simulink model "HydroPower"  (R2024b)
settings: Solver=ode4  StartTime=0.0  StopTime=200  FixedStep=0.001  RelTol=1e-3
values from neighbouring files (symbols this model uses):
  Af = 0.01    [Data__MOTOR.m]    (also in Generator_Data.m = 0.0001; Generator_Datatest.m)
  Bf = 0.0002    [Data__MOTOR.m]    (also in Generator_Data.m = 2e-05; Generator_Datatest.m)
  Cr = 0    [Generator_Data.m]
  CurrentFaultSwitch = 0    [Data__MOTOR.m]    (also in Generator_Data.m = 1; Generator_Datatest.m)
  f = 0.001    [Data__MOTOR.m]    (also in Generator_Data.m = 0)
  J = 0.0012    [Data__MOTOR.m]    (also in Generator_Data.m = 0.263; Generator_Datatest.m = 0.263)
  Ld = 1.4e-3+L_charge    (= 0.0014)    [Generator_Data.m]    (also in Generator_Datatest.m = 0.0231)
  Lq = 2.8e-3+L_charge    (= 0.0028)    [Generator_Data.m]    (also in Generator_Datatest.m = 0.0231)
  P = 4    [Generator_Data.m]    (also in Generator_Datatest.m = 3)
  Phif = 0.8    [Generator_Data.m]
  rate_noise_i = 0.02*In    (= 0.22)    [Data__MOTOR.m]    (also in Generator_Data.m = 0.02; Generator_Datatest.m)
  rate_noise_w = 0.02*Wn    (= 2.96)    [Data__MOTOR.m]    (also in Generator_Data.m = 0.002; Generator_Datatest.m)
  Rs = 0.6+R_charge    (= 0.6)    [Generator_Data.m]    (also in Generator_Datatest.m = 0.48)
  StartStop = 0    [Data__MOTOR.m]    (also in Generator_Data.m; Generator_Datatest.m)
  Te = 0.1    [Data__MOTOR.m]    (also in Generator_Data.m = 1; Generator_Datatest.m)
  Vd = 0    [Generator_Data.m]
  VelocityFaultSwitch = 0    [Data__MOTOR.m]    (also in Generator_Data.m = 1; Generator_Datatest.m)
  Vq = 0    [Generator_Data.m]
  wm = 2*pi*50/P    (= 78.5398163397)    [Generator_Data.m]
undefined symbols (not defined in the file or in its folder): dspblkCoreblockFVToolHelper, gcbh
libraries: SignalEditorBlockLib x3
(part 3 of 3)

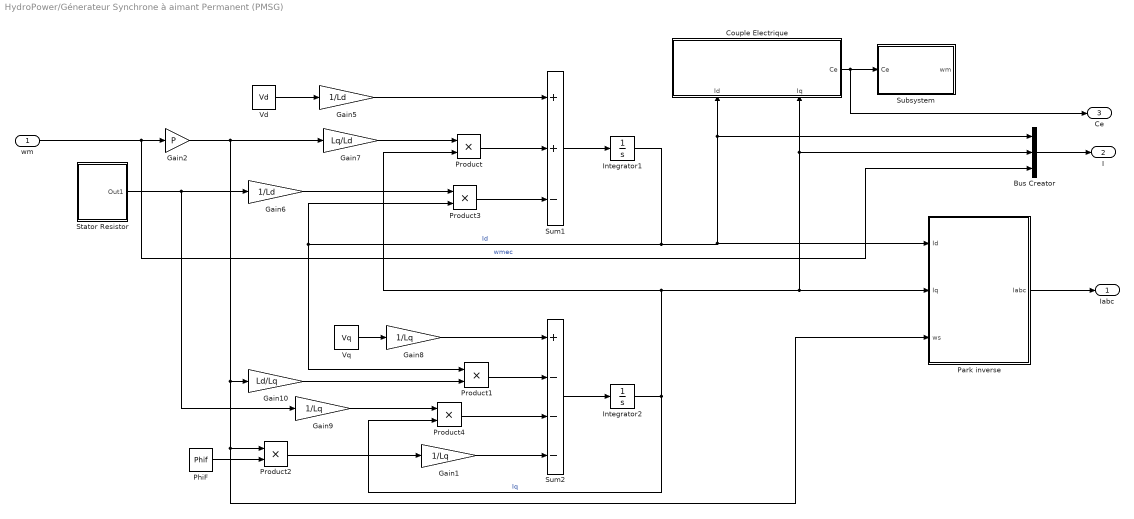
== system HydroPower/Génerateur Synchrone à aimant Permanent (PMSG) ==
  "wm " : Inport
  Bus Creator : BusCreator  Inputs=3
  Couple Electrique : Subsystem
      settings: PortSchema="{\"entries\":[{\"content\":{\"sides\":[{\"content\":{},\"type\":\"ConnectorPlacement.EquallySpacedRectSide\",\"uuid\":\"d44e9c0e-d895-4bd1-ae10-379ff1646526\"},{\"content\":{\"connectorIds\":[\"Out1\"],\"side\":\"RIGHT\"},\"type\":\"ConnectorPlacement.EquallySpacedRectSide\",\"uuid\":\"f5af5393-6c68-4e11-bc58-eb62e675a1fd\"},{\"content\":{\"side\":\"TOP\"},\"type\":\"ConnectorPlacement.EquallySpacedRectSide\",\"uuid\":\"8c0d084d-7b17-4a57-bb76-f17d1f7247d1\"},{\"content\":{\"connectorIds\":[\"In1\",\"In2\"],\"side\":\"BOTTOM\"},\"type\":\"ConnectorPlacement.EquallySpacedRectSide\",\"uuid\":\"33e36c13-4871-4cd2-bb8a-e9a834d32846\"}]},\"type\":\"ConnectorPlacement.EquallySpacedConnector\",\"uuid\":\"c176d3db-292c-4956-9d3a-590d4025293f\"}],\"packageUris\":[\"http://schema.mathworks.com/mf0/Connector/R2020b\"],\"version\":\"1.0\"}"
      mask Display:
      | disp('Couple électrique')
      | port_label('input', 1, 'Id');
      | port_label('input', 2, 'Iq');
      | port_label('output', 1, 'Ce');
  Gain1 : Gain  Gain=1/Lq
  Gain10 : Gain  Gain=Ld/Lq
  Gain2 : Gain  Gain=P
  Gain5 : Gain  Gain=1/Ld
  Gain6 : Gain  Gain=1/Ld
  Gain7 : Gain  Gain=Lq/Ld
  Gain8 : Gain  Gain=1/Lq
  Gain9 : Gain  Gain=1/Lq
  Integrator1 : Integrator
  Integrator2 : Integrator
  Park inverse : Subsystem
      mask Display:
      | color('black');
      | disp('Park\n Inverse')
      | %color('yellow');
      | 
      | port_label('input', 1, 'I_{d}','texmode','on');
      | port_label('input', 2, 'I_{q}','texmode','on');
      | port_label('input', 3, '\omega_{s}','texmode','on');
      | 
      | %color('green');
      | 
      | port_label('output', 1, 'I_{abc}','texmode','on');
  PhiF : Constant  Value=Phif
  Product{,1..4} (5 alike) : Product
  Stator Resistor : Subsystem
      mask Display: disp('Stator \n Resistor')
  Subsystem : Subsystem
  Sum1 : Sum  Inputs=++-
  Sum2 : Sum  Inputs=+---
  Vd : Constant  Value=Vd
  Vq : Constant  Value=Vq
  "Iabc " : Outport
  I : Outport  Port=2
  Ce : Outport  Port=3
  wires:
  Park inverse/1(Iabc) -> "Iabc "/1
  Vd/1 -> Gain5/1
  Gain5/1 -> Sum1/1
  Integrator2/1 -> Product/2, Couple Electrique/2(Iq), Bus Creator/2, Park inverse/2(Iq), Product4/2  "Iq"
  Sum1/1 -> Integrator1/1
  Sum2/1 -> Integrator2/1
  Vq/1 -> Gain8/1
  Gain8/1 -> Sum2/1
  Integrator1/1 -> Product3/2, Product1/1, Couple Electrique/1(Id), Bus Creator/1, Park inverse/1(Id)  "Id"
  Gain10/1 -> Product1/2
  PhiF/1 -> Product2/2
  Product2/1 -> Gain1/1
  Product/1 -> Sum1/2
  Gain1/1 -> Sum2/4
  Product1/1 -> Sum2/2
  "wm "/1 -> Bus Creator/3, Gain2/1  "wmec"
  Gain2/1 -> Park inverse/3(ws), Product2/1, Gain10/1, Gain7/1
  Gain7/1 -> Product/1
  Stator Resistor/1(Out1) -> Gain9/1, Gain6/1
  Product3/1 -> Sum1/3
  Gain6/1 -> Product3/1
  Product4/1 -> Sum2/3
  Gain9/1 -> Product4/1
  Couple Electrique/1(Ce) -> Ce/1, Subsystem/1(Ce)
  Bus Creator/1 -> I/1

== system HydroPower/Turbine ==
  wmec : Constant  Value=wm  SampleTime=-1
  "wmec " : Outport
  wires:
  wmec/1 -> "wmec "/1

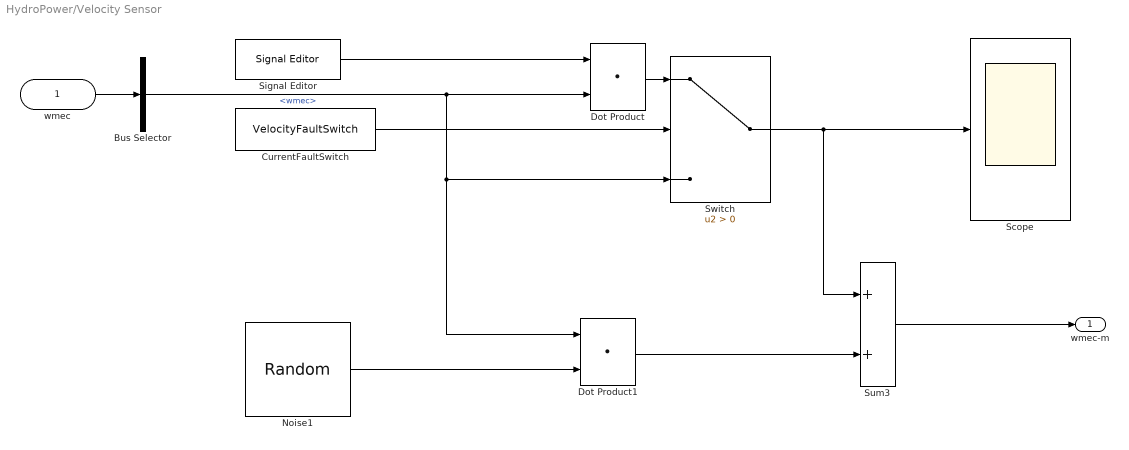
== system HydroPower/Velocity Sensor ==
  wmec : Inport
  Bus Selector : BusSelector  OutputSignals=wmec
  CurrentFaultSwitch : Constant  Value=VelocityFaultSwitch  SampleTime=-1
  Dot Product : DotProduct  OutDataTypeStr=Inherit: Inherit via internal rule
  Dot Product1 : DotProduct  OutDataTypeStr=Inherit: Inherit via internal rule
  Noise1 : UniformRandomNumber  Minimum=-rate_noise_w  Maximum=+rate_noise_w  SampleTime=0.01
  Scope : Scope
  Signal Editor : SignalEditorBlockLib/Signal Editor  FileName=VelocityFault.mat  ActiveScenario=ChuteVelocite  ActiveSignal=Fault  IsBus=off  OutputBusObjectStr=Bus: BusObject  SampleTime=0  Interpolate=off  ZeroCross=off  OutputAfterFinalValue=Setting to zero  Unit=inherit  PreserveSignalName=on  ApplySigPropsToAllScenarios=on  ApplySigPropsToAllSignals=off
  Sum3 : Sum  InputSameDT=on  SaturateOnIntegerOverflow=on  OutDataTypeStr=Inherit: Same as first input
  Switch : Switch  Criteria=u2 > Threshold  SaturateOnIntegerOverflow=off  InputSameDT=off
  wmec-m : Outport  VectorParamsAs1DForOutWhenUnconnected=off
  wires:
  Sum3/1 -> wmec-m/1
  Switch/1 -> Scope/1, Sum3/1
  CurrentFaultSwitch/1 -> Switch/2
  Noise1/1 -> Dot Product1/2
  Bus Selector/1 -> Dot Product1/1, Switch/3, Dot Product/2  "<wmec>"
  Signal Editor/1 -> Dot Product/1
  Dot Product1/1 -> Sum3/2
  Dot Product/1 -> Switch/1
  wmec/1 -> Bus Selector/1

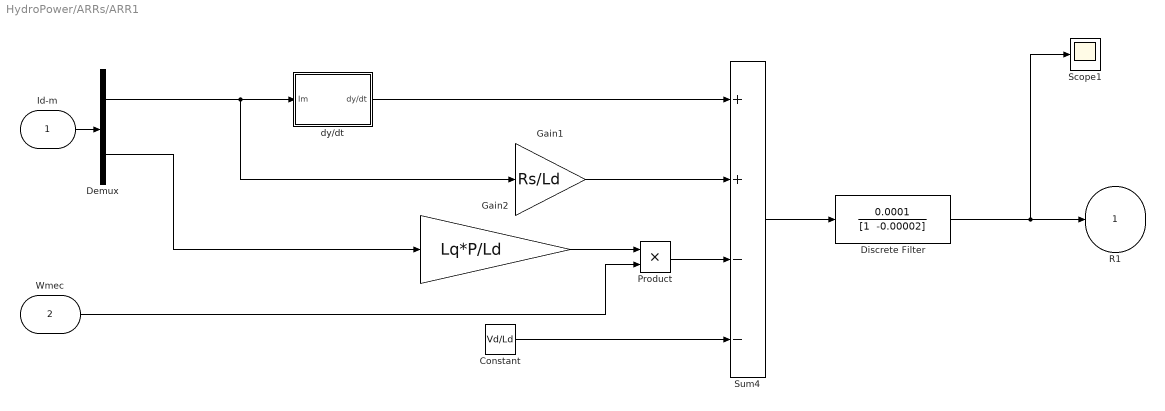
== system HydroPower/ARRs/ARR1 ==
  Id-m : Inport
  Wmec : Inport  Port=2
  Constant : Constant  Value=Vd/Ld
  Demux : Demux  Outputs=2
  Discrete Filter : DiscreteFilter  LoadFcn=dspblkCoreblockFVToolHelper(gcbh,'load');  Numerator=0.0001  Denominator="[1  -0.00002]"  SampleTime=0.001  a0EqualsOne=on
      settings: CopyFcn=dspblkCoreblockFVToolHelper(gcbh,'copy');  DeleteFcn=dspblkCoreblockFVToolHelper(gcbh,'close');  ModelCloseFcn=dspblkCoreblockFVToolHelper(gcbh,'close');  PreSaveFcn=dspblkCoreblockFVToolHelper(gcbh,'presave');  PostSaveFcn=dspblkCoreblockFVToolHelper(gcbh,'postsave');  CloseFcn=dspblkCoreblockFVToolHelper(gcbh,'close');
  Gain1 : Gain  Gain=Rs/Ld
  Gain2 : Gain  Gain=Lq*P/Ld
  Product : Product
  Scope1 : Scope
  Sum4 : Sum  Inputs=++--
  dy/dt : Subsystem
  R1 : Outport  VectorParamsAs1DForOutWhenUnconnected=off
  wires:
  Gain1/1 -> Sum4/2
  Demux/1 -> dy/dt/1(Im), Gain1/1
  Id-m/1 -> Demux/1
  Demux/2 -> Gain2/1
  Gain2/1 -> Product/1
  Product/1 -> Sum4/3
  Constant/1 -> Sum4/4
  Sum4/1 -> Discrete Filter/1
  Discrete Filter/1 -> Scope1/1, R1/1
  Wmec/1 -> Product/2
  dy/dt/1(dy/dt) -> Sum4/1

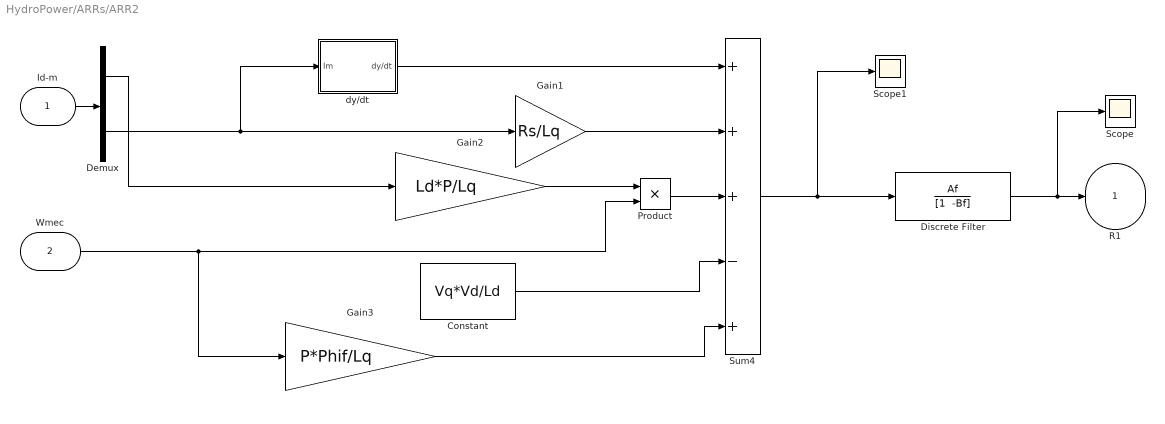
== system HydroPower/ARRs/ARR2 ==
  Id-m : Inport
  Wmec : Inport  Port=2
  Constant : Constant  Value=Vq*Vd/Ld
  Demux : Demux  Outputs=2
  Discrete Filter : DiscreteFilter  LoadFcn=dspblkCoreblockFVToolHelper(gcbh,'load');  Numerator=Af  Denominator="[1  -Bf]"  SampleTime=0.01  a0EqualsOne=on
      settings: CopyFcn=dspblkCoreblockFVToolHelper(gcbh,'copy');  DeleteFcn=dspblkCoreblockFVToolHelper(gcbh,'close');  ModelCloseFcn=dspblkCoreblockFVToolHelper(gcbh,'close');  PreSaveFcn=dspblkCoreblockFVToolHelper(gcbh,'presave');  PostSaveFcn=dspblkCoreblockFVToolHelper(gcbh,'postsave');  CloseFcn=dspblkCoreblockFVToolHelper(gcbh,'close');
  Gain1 : Gain  Gain=Rs/Lq
  Gain2 : Gain  Gain=Ld*P/Lq
  Gain3 : Gain  Gain=P*Phif/Lq
  Product : Product
  Scope : Scope
  Scope1 : Scope
  Sum4 : Sum  Inputs=+++-+
  dy/dt : Subsystem
  R1 : Outport  VectorParamsAs1DForOutWhenUnconnected=off
  wires:
  Discrete Filter/1 -> Scope/1, R1/1
  Sum4/1 -> Scope1/1, Discrete Filter/1
  Constant/1 -> Sum4/4
  Wmec/1 -> Gain3/1, Product/2
  Product/1 -> Sum4/3
  Gain2/1 -> Product/1
  Id-m/1 -> Demux/1
  dy/dt/1(dy/dt) -> Sum4/1
  Demux/2 -> dy/dt/1(Im), Gain1/1
  Gain1/1 -> Sum4/2
  Gain3/1 -> Sum4/5
  Demux/1 -> Gain2/1

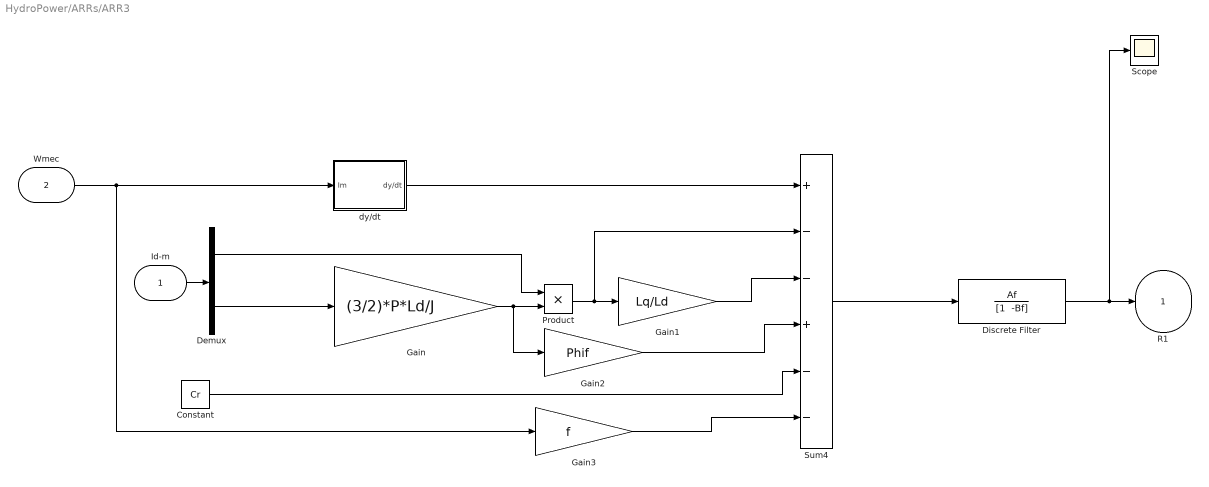
== system HydroPower/ARRs/ARR3 ==
  Id-m : Inport
  Wmec : Inport  Port=2
  Constant : Constant  Value=Cr
  Demux : Demux  Outputs=2
  Discrete Filter : DiscreteFilter  LoadFcn=dspblkCoreblockFVToolHelper(gcbh,'load');  Numerator=Af  Denominator="[1  -Bf]"  SampleTime=0.01  a0EqualsOne=on
      settings: CopyFcn=dspblkCoreblockFVToolHelper(gcbh,'copy');  DeleteFcn=dspblkCoreblockFVToolHelper(gcbh,'close');  ModelCloseFcn=dspblkCoreblockFVToolHelper(gcbh,'close');  PreSaveFcn=dspblkCoreblockFVToolHelper(gcbh,'presave');  PostSaveFcn=dspblkCoreblockFVToolHelper(gcbh,'postsave');  CloseFcn=dspblkCoreblockFVToolHelper(gcbh,'close');
  Gain : Gain  Gain=(3/2)*P*Ld/J
  Gain1 : Gain  Gain=Lq/Ld
  Gain2 : Gain  Gain=Phif
  Gain3 : Gain  Gain=f
  Product : Product
  Scope : Scope
  Sum4 : Sum  Inputs=+--+--
  dy/dt : Subsystem
  R1 : Outport  VectorParamsAs1DForOutWhenUnconnected=off
  wires:
  Id-m/1 -> Demux/1
  Gain1/1 -> Sum4/3
  Sum4/1 -> Discrete Filter/1
  Discrete Filter/1 -> Scope/1, R1/1
  Wmec/1 -> dy/dt/1(Im), Gain3/1
  dy/dt/1(dy/dt) -> Sum4/1
  Demux/2 -> Gain/1
  Gain/1 -> Gain2/1, Product/2
  Demux/1 -> Product/1
  Product/1 -> Sum4/2, Gain1/1
  Gain2/1 -> Sum4/4
  Constant/1 -> Sum4/5
  Gain3/1 -> Sum4/6

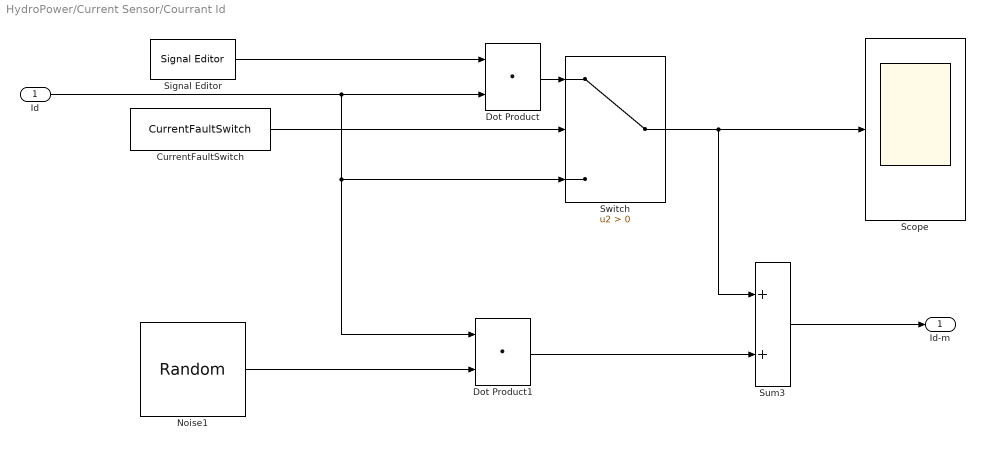
== system HydroPower/Current Sensor/Courrant Id ==
  Id : Inport
  CurrentFaultSwitch : Constant  Value=CurrentFaultSwitch  SampleTime=-1
  Dot Product : DotProduct  OutDataTypeStr=Inherit: Inherit via internal rule
  Dot Product1 : DotProduct  OutDataTypeStr=Inherit: Inherit via internal rule
  Noise1 : UniformRandomNumber  Minimum=-rate_noise_i  Maximum=+rate_noise_i  SampleTime=0.01
  Scope : Scope
  Signal Editor : SignalEditorBlockLib/Signal Editor  FileName=CurrentFault.mat  ActiveScenario=ChuteCourant  ActiveSignal=Fault  IsBus=off  OutputBusObjectStr=Bus: BusObject  SampleTime=0  Interpolate=off  ZeroCross=off  OutputAfterFinalValue=Setting to zero  Unit=inherit  PreserveSignalName=on  ApplySigPropsToAllScenarios=on  ApplySigPropsToAllSignals=off
  Sum3 : Sum  InputSameDT=on  SaturateOnIntegerOverflow=on  OutDataTypeStr=Inherit: Same as first input
  Switch : Switch  Criteria=u2 > Threshold  SaturateOnIntegerOverflow=off  InputSameDT=off
  Id-m : Outport
  wires:
  Signal Editor/1 -> Dot Product/1
  Id/1 -> Switch/3, Dot Product1/1, Dot Product/2
  Sum3/1 -> Id-m/1
  CurrentFaultSwitch/1 -> Switch/2
  Switch/1 -> Sum3/1, Scope/1
  Dot Product/1 -> Switch/1
  Noise1/1 -> Dot Product1/2
  Dot Product1/1 -> Sum3/2

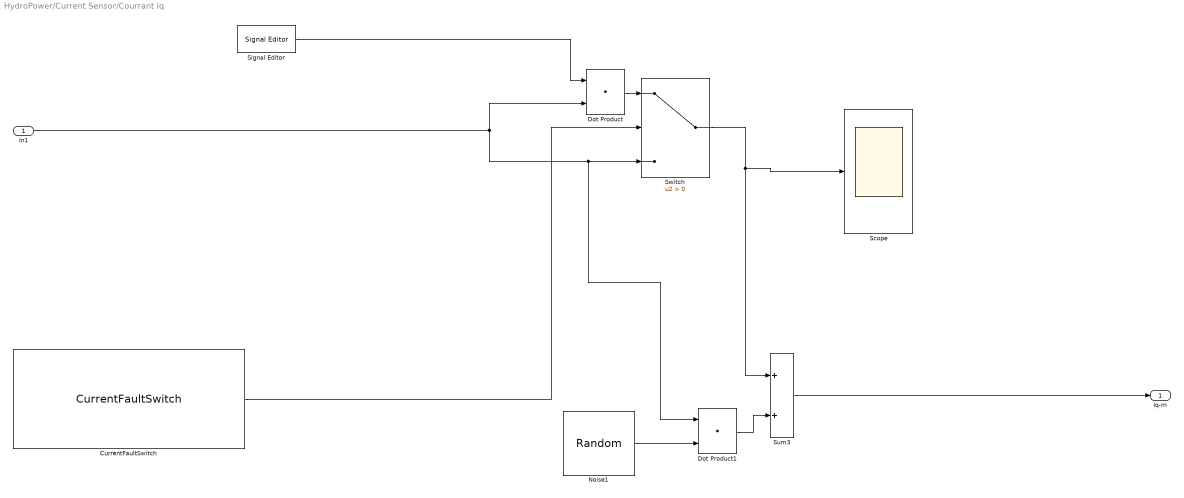
== system HydroPower/Current Sensor/Courrant Iq ==
  In1 : Inport
  CurrentFaultSwitch : Constant  Value=CurrentFaultSwitch  SampleTime=-1
  Dot Product : DotProduct  OutDataTypeStr=Inherit: Inherit via internal rule
  Dot Product1 : DotProduct  OutDataTypeStr=Inherit: Inherit via internal rule
  Noise1 : UniformRandomNumber  Minimum=-rate_noise_i  Maximum=+rate_noise_i  SampleTime=0.01
  Scope : Scope
  Signal Editor : SignalEditorBlockLib/Signal Editor  FileName=CurrentFault.mat  ActiveScenario=ChuteCourant  ActiveSignal=Fault  IsBus=off  OutputBusObjectStr=Bus: BusObject  SampleTime=0  Interpolate=off  ZeroCross=off  OutputAfterFinalValue=Setting to zero  Unit=inherit  PreserveSignalName=on  ApplySigPropsToAllScenarios=on  ApplySigPropsToAllSignals=off
  Sum3 : Sum  InputSameDT=on  SaturateOnIntegerOverflow=on  OutDataTypeStr=Inherit: Same as first input
  Switch : Switch  Criteria=u2 > Threshold  SaturateOnIntegerOverflow=off  InputSameDT=off
  Iq-m : Outport
  wires:
  Dot Product1/1 -> Sum3/2
  Noise1/1 -> Dot Product1/2
  Dot Product/1 -> Switch/1
  Switch/1 -> Scope/1, Sum3/1
  CurrentFaultSwitch/1 -> Switch/2
  Sum3/1 -> Iq-m/1
  In1/1 -> Dot Product/2, Switch/3, Dot Product1/1
  Signal Editor/1 -> Dot Product/1

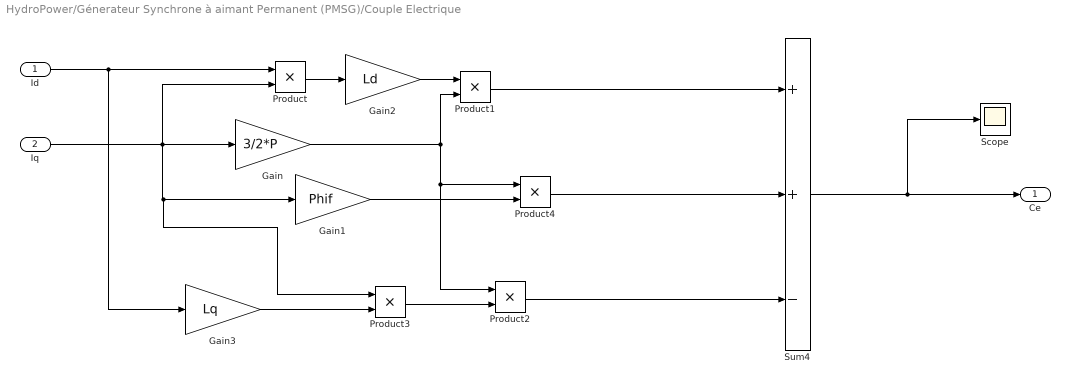
== system HydroPower/Génerateur Synchrone à aimant Permanent (PMSG)/Couple Electrique ==
  Id : Inport
  Iq : Inport  Port=2
  Gain : Gain  Gain=3/2*P
  Gain1 : Gain  Gain=Phif
  Gain2 : Gain  Gain=Ld
  Gain3 : Gain  Gain=Lq
  Product{,1..4} (5 alike) : Product
  Scope : Scope
  Sum4 : Sum  Inputs=++-
  Ce : Outport
  wires:
  Sum4/1 -> Scope/1, Ce/1
  Iq/1 -> Product/2, Product3/1, Gain1/1, Gain/1
  Product/1 -> Gain2/1
  Gain2/1 -> Product1/1
  Gain/1 -> Product2/1, Product4/1, Product1/2
  Product1/1 -> Sum4/1
  Id/1 -> Gain3/1, Product/1
  Gain1/1 -> Product4/2
  Product4/1 -> Sum4/2
  Product2/1 -> Sum4/3
  Product3/1 -> Product2/2
  Gain3/1 -> Product3/2

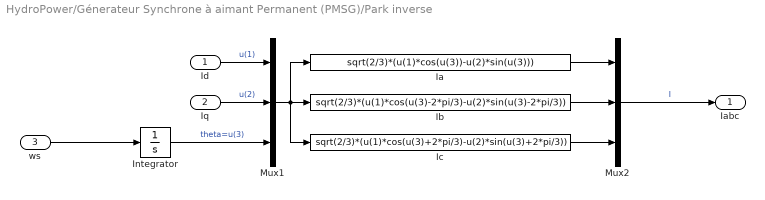
== system HydroPower/Génerateur Synchrone à aimant Permanent (PMSG)/Park inverse ==
  Id : Inport
  Iq : Inport  Port=2
  ws : Inport  Port=3
  Ia : Fcn  Expr=sqrt(2/3)*(u(1)*cos(u(3))-u(2)*sin(u(3)))
  Ib : Fcn  Expr=sqrt(2/3)*(u(1)*cos(u(3)-2*pi/3)-u(2)*sin(u(3)-2*pi/3))
  Ic : Fcn  Expr=sqrt(2/3)*(u(1)*cos(u(3)+2*pi/3)-u(2)*sin(u(3)+2*pi/3))
  Integrator : Integrator
  Mux1 : Mux  Inputs=3
  Mux2 : Mux  Inputs=3
  Iabc : Outport
  wires:
  ws/1 -> Integrator/1
  Integrator/1 -> Mux1/3  "theta=u(3)"
  Id/1 -> Mux1/1  "u(1)"
  Iq/1 -> Mux1/2  "u(2)"
  Ia/1 -> Mux2/1
  Ic/1 -> Mux2/3
  Ib/1 -> Mux2/2
  Mux2/1 -> Iabc/1  "I"
  Mux1/1 -> Ia/1, Ic/1, Ib/1

== system HydroPower/Génerateur Synchrone à aimant Permanent (PMSG)/Stator Resistor ==
  Constant : Constant  Value=Rs
  Out1 : Outport
  wires:
  Constant/1 -> Out1/1

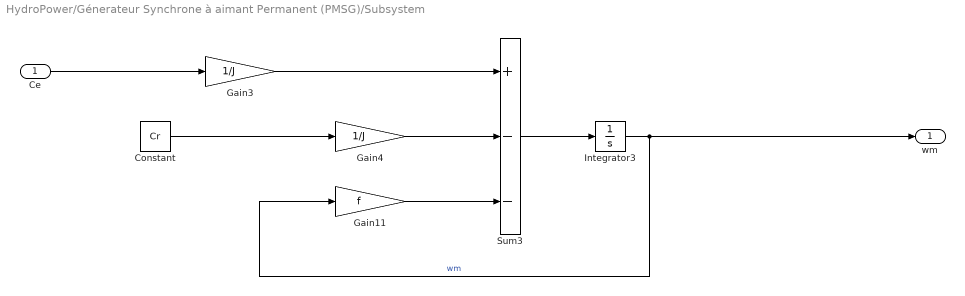
== system HydroPower/Génerateur Synchrone à aimant Permanent (PMSG)/Subsystem ==
  Ce : Inport
  Constant : Constant  Value=Cr
  Gain11 : Gain  Gain=f
  Gain3 : Gain  Gain=1/J
  Gain4 : Gain  Gain=1/J
  Integrator3 : Integrator
  Sum3 : Sum  Inputs=+--
  wm : Outport
  wires:
  Gain3/1 -> Sum3/1
  Gain11/1 -> Sum3/3
  Gain4/1 -> Sum3/2
  Constant/1 -> Gain4/1
  Integrator3/1 -> wm/1, Gain11/1  "wm"
  Sum3/1 -> Integrator3/1
  Ce/1 -> Gain3/1

== system HydroPower/ARRs/ARR1/dy//dt ==
  note: dY/dt= ((y(k)-y(k-1))/Te
  note: Y(k)
  note: Y(k-1
  Im : Inport
  Delay : Delay  DelayLength=1  SampleTime=Te
  Gain2 : Gain  Gain=1/10
  Sum1 : Sum  Inputs=+-
  dy/dt : Outport  VectorParamsAs1DForOutWhenUnconnected=off
  wires:
  Gain2/1 -> dy/dt/1
  Sum1/1 -> Gain2/1
  Delay/1 -> Sum1/2
  Im/1 -> Delay/1, Sum1/1

== system HydroPower/ARRs/ARR2/dy//dt ==
  note: dY/dt= ((y(k)-y(k-1))/Te
  note: Y(k)
  note: Y(k-1
  Im : Inport
  Delay : Delay  DelayLength=1  SampleTime=Te
  Gain2 : Gain  Gain=1/10
  Sum1 : Sum  Inputs=+-
  dy/dt : Outport  VectorParamsAs1DForOutWhenUnconnected=off
  wires:
  Gain2/1 -> dy/dt/1
  Sum1/1 -> Gain2/1
  Delay/1 -> Sum1/2
  Im/1 -> Delay/1, Sum1/1

== system HydroPower/ARRs/ARR3/dy//dt ==
  note: dY/dt= ((y(k)-y(k-1))/Te
  note: Y(k)
  note: Y(k-1
  Im : Inport
  Delay : Delay  DelayLength=1  SampleTime=Te
  Gain2 : Gain  Gain=1/10
  Sum1 : Sum  Inputs=+-
  dy/dt : Outport  VectorParamsAs1DForOutWhenUnconnected=off
  wires:
  Gain2/1 -> dy/dt/1
  Sum1/1 -> Gain2/1
  Delay/1 -> Sum1/2
  Im/1 -> Delay/1, Sum1/1
